simulink model "control_y_sistemas_0"  (R2023a)
settings: Solver=VariableStepAuto  StartTime=0.0  StopTime=sim_end_time  RelTol=1e-3
values from neighbouring files (symbols this model uses):
  alpha_cu = 3.9 *10^-3    (= 0.0039)    [BLDC_Motor_params_03.m]    (also in DC_Motor_params_01.m; DC_Motor_params_02.m; DC_Motor_params_04.m; DC_Motor_params_05.m)
  b_m1 = .01    (= 0.01)    [DC_Motor_params_01.m]
  C_t1 = 19.57    [DC_Motor_params_01.m]
  J_eq1 = J_1 + 1/8 * m_1 * d_1^2 / r_1^2    [DC_Motor_params_01.m]
  k_e1 = 0.25    [DC_Motor_params_01.m]
  k_t1 = 0.25    [DC_Motor_params_01.m]
  L_a1 = 7.5*10^-3    (= 0.0075)    [DC_Motor_params_01.m]
  r_1 = 25    [DC_Motor_params_01.m]
  r_a1_20 = 0.5    [DC_Motor_params_01.m]
  res_term_1 = 9.58    [DC_Motor_params_01.m]
  theta_m1_0 = 0    [verify_cl_pid.m]    (also in verify_ol_model.m)
settings Model: Creator=Usuario  LastModifiedBy=Usuario
settings DataIOCC: ExternalInput=[sim_t sim_data_in]  LoadExternalInput=on

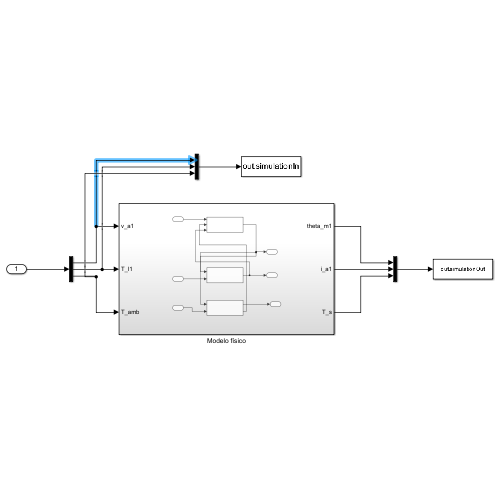
[thumbnail: Simulink's stored preview of the top-level diagram]
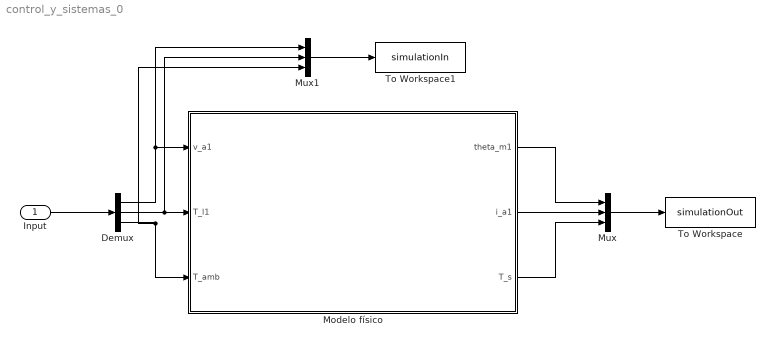
== system control_y_sistemas_0 ==
  Input : Inport
  Demux : Demux  Outputs=3
  Modelo físico : Subsystem
  Mux : Mux  Inputs=3
  Mux1 : Mux  Inputs=3
  To Workspace : ToWorkspace  VariableName=simulationOut  SaveFormat=Timeseries  SampleTime=-1
  To Workspace1 : ToWorkspace  VariableName=simulationIn  SaveFormat=Timeseries  SampleTime=-1
  wires:
  Input/1 -> Demux/1
  Demux/1 -> Mux1/1, Modelo físico/1(v_a1)
  Demux/2 -> Mux1/2, Modelo físico/2(T_l1)
  Modelo físico/1(theta_m1) -> Mux/1
  Mux1/1 -> To Workspace1/1
  Mux/1 -> To Workspace/1
  Modelo físico/2(i_a1) -> Mux/2
  Demux/3 -> Mux1/3, Modelo físico/3(T_amb)
  Modelo físico/3(T_s) -> Mux/3

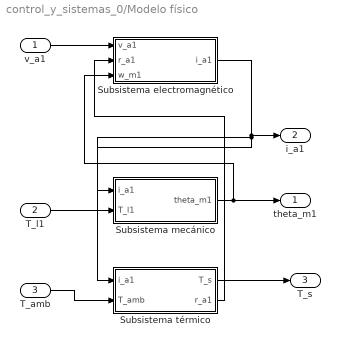
== system control_y_sistemas_0/Modelo físico ==
  v_a1 : Inport
  T_l1 : Inport  Port=2
  T_amb : Inport  Port=3
  Subsistema electromagnético : Subsystem
  Subsistema mecánico : Subsystem
  Subsistema térmico : Subsystem
  theta_m1 : Outport
  i_a1 : Outport  Port=2
  T_s : Outport  Port=3
  wires:
  Subsistema mecánico/1(theta_m1) -> theta_m1/1, Subsistema electromagnético/3(w_m1)
  Subsistema electromagnético/1(i_a1) -> Subsistema térmico/1(i_a1), Subsistema mecánico/1(i_a1), i_a1/1
  v_a1/1 -> Subsistema electromagnético/1(v_a1)
  T_l1/1 -> Subsistema mecánico/2(T_l1)
  T_amb/1 -> Subsistema térmico/2(T_amb)
  Subsistema térmico/1(T_s) -> T_s/1
  Subsistema térmico/2(r_a1) -> Subsistema electromagnético/2(r_a1)

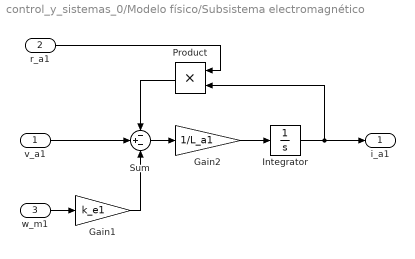
== system control_y_sistemas_0/Modelo físico/Subsistema electromagnético ==
  v_a1 : Inport
  r_a1 : Inport  Port=2
  w_m1 : Inport  Port=3
  Gain1 : Gain  Gain=k_e1
  Gain2 : Gain  Gain=1/L_a1
  Integrator : Integrator
  Product : Product
  Sum : Sum  Inputs=-+-
  i_a1 : Outport
  wires:
  v_a1/1 -> Sum/2
  Integrator/1 -> Product/2, i_a1/1
  Product/1 -> Sum/1
  w_m1/1 -> Gain1/1
  Gain1/1 -> Sum/3
  Sum/1 -> Gain2/1
  Gain2/1 -> Integrator/1
  r_a1/1 -> Product/1

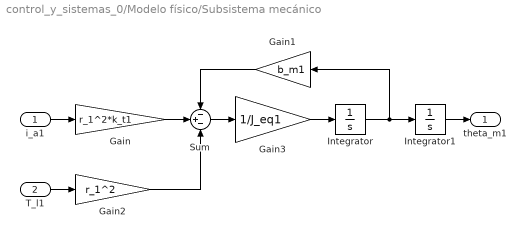
== system control_y_sistemas_0/Modelo físico/Subsistema mecánico ==
  i_a1 : Inport
  T_l1 : Inport  Port=2
  Gain : Gain  Gain=r_1^2*k_t1
  Gain1 : Gain  Gain=b_m1
  Gain2 : Gain  Gain=r_1^2
  Gain3 : Gain  Gain=1/J_eq1
  Integrator : Integrator
  Integrator1 : Integrator  InitialCondition=theta_m1_0
  Sum : Sum  Inputs=-+-
  theta_m1 : Outport
  wires:
  i_a1/1 -> Gain/1
  Gain/1 -> Sum/2
  Integrator/1 -> Gain1/1, Integrator1/1
  Gain1/1 -> Sum/1
  T_l1/1 -> Gain2/1
  Gain2/1 -> Sum/3
  Gain3/1 -> Integrator/1
  Sum/1 -> Gain3/1
  Integrator1/1 -> theta_m1/1

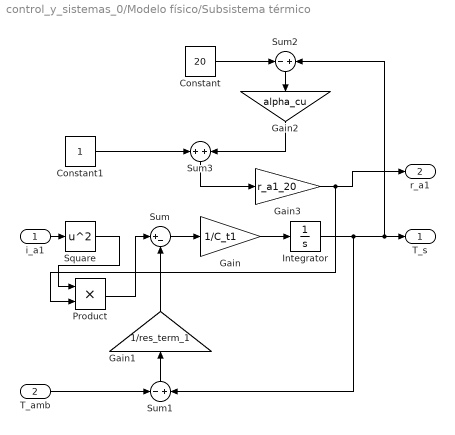
== system control_y_sistemas_0/Modelo físico/Subsistema térmico ==
  i_a1 : Inport
  T_amb : Inport  Port=2
  Constant : Constant  Value=20
  Constant1 : Constant
  Gain : Gain  Gain=1/C_t1
  Gain1 : Gain  Gain=1/res_term_1
  Gain2 : Gain  Gain=alpha_cu
  Gain3 : Gain  Gain=r_a1_20
  Integrator : Integrator
  Product : Product
  Square : Math  Operator=square
  Sum : Sum  Inputs=|+-
  Sum1 : Sum  Inputs=-|+
  Sum2 : Sum  Inputs=-|+
  Sum3 : Sum  Inputs=+|+
  T_s : Outport
  r_a1 : Outport  Port=2
  wires:
  i_a1/1 -> Square/1
  Sum/1 -> Gain/1
  Gain/1 -> Integrator/1
  Integrator/1 -> Sum1/2, Sum2/2, T_s/1
  Gain1/1 -> Sum/2
  Sum1/1 -> Gain1/1
  T_amb/1 -> Sum1/1
  Constant/1 -> Sum2/1
  Sum2/1 -> Gain2/1
  Constant1/1 -> Sum3/1
  Gain2/1 -> Sum3/2
  Sum3/1 -> Gain3/1
  Gain3/1 -> Product/2, r_a1/1
  Square/1 -> Product/1
  Product/1 -> Sum/1
